simulink model "Control_System_6"  (R2018a)
settings: Solver=VariableStepAuto  StartTime=0.0  StopTime=30.0  RelTol=1e-3
libraries: dspsrcs4 x2
settings Model: Creator=bhanubhandari  LastModifiedBy=bhanubhandari

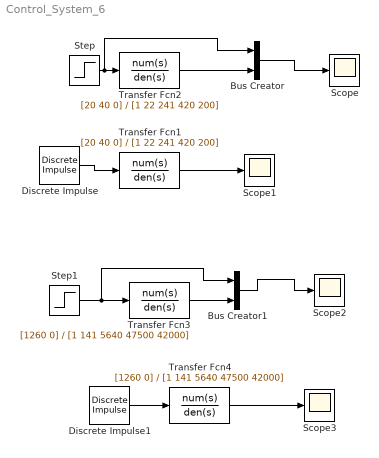
== system Control_System_6 ==
  Bus Creator : BusCreator  Inputs=2
  Bus Creator1 : BusCreator  Inputs=2
  Discrete Impulse : dspsrcs4/Discrete  Impulse  Delay=0  SampleTime=1  FrameSample=1  OutputFrames=off  dataType=double  isSigned=on  wordLen=16  udDataType=sfix(16)  fracBitsMode=Best precision  numFracBits=15  OutDataTypeStr=double  LastOutDataTypeStr=double
  Discrete Impulse1 : dspsrcs4/Discrete  Impulse  Delay=0  SampleTime=1  FrameSample=1  OutputFrames=off  dataType=double  isSigned=on  wordLen=16  udDataType=sfix(16)  fracBitsMode=Best precision  numFracBits=15  OutDataTypeStr=double  LastOutDataTypeStr=double
  Scope{,1..3} (4 alike) : Scope
  Step : Step  SampleTime=0
  Step1 : Step  SampleTime=0
  Transfer Fcn1 : TransferFcn  Numerator=[20 40 0]  Denominator=[1 22 241 420 200]
  Transfer Fcn2 : TransferFcn  Numerator=[20 40 0]  Denominator=[1 22 241 420 200]
  Transfer Fcn3 : TransferFcn  Numerator=[1260 0]  Denominator=[1 141 5640 47500 42000]
  Transfer Fcn4 : TransferFcn  Numerator=[1260 0]  Denominator=[1 141 5640 47500 42000]
  wires:
  Step/1 -> Bus Creator/1, Transfer Fcn2/1
  Transfer Fcn2/1 -> Bus Creator/2
  Bus Creator/1 -> Scope/1
  Discrete Impulse/1 -> Transfer Fcn1/1
  Transfer Fcn1/1 -> Scope1/1
  Transfer Fcn3/1 -> Bus Creator1/2
  Step1/1 -> Bus Creator1/1, Transfer Fcn3/1
  Bus Creator1/1 -> Scope2/1
  Discrete Impulse1/1 -> Transfer Fcn4/1
  Transfer Fcn4/1 -> Scope3/1
